simulink library "VRU_MC_Search"  (Simulink 8.1)
settings: Solver=ode1  StartTime=0.0  StopTime=Inf  FixedStep=0.001  RelTol=1e-3
PostLoadFcn:
  | , if any(exist('dsrtsu_mdlpostloadfcn', 'file') == [2, 3, 6]), try dsrtsu_mdlpostloadfcn('Execute', bdroot); catch fprintf('Error in PostLoadFcn (dsrtsu_mdlpostloadfcn) for model "%s":\n %s\n', bdroot, lasterr); end, end,
undefined symbols (not defined in the file or in its folder): KIFO_VRUExistProbLimit_num, ZERO_INT
settings Model: DSRTSU_INTERNAL_RTI_VER=450  DSRTSU_INTERNAL_RTI_TYPE=rti1401  RTICANMMDATA=struct('GeneralSetupData',struct('modelroot','D:\PROJECTS\HAITEC\TAIWAN_HAITEC_SVN\trunk\AdasDragon\software\sw_development\arch\app\ifo','generalsettings',struct('filesettings',struct('destfolder',struct('Name','RTICANMM_FILES','Check',1),'buildfolder',struct('Name','.','Check',1),'AbsDestfolder',struct('Name','D:\PROJECTS\HAITEC\TAIWAN_HAITEC_SVN\trunk\AdasDragon\software\sw_development\arch\app\ifo\RTICANMM_FILES'),'AbsBuildfolder',struct('Name','D:\PROJECTS\HAITEC\TAIWAN_HAITEC_SVN\trunk\AdasDragon\software\sw_development\arch\app\ifo'))),'options',struct('addpaths',1,'rmpaths',1,'addtrcexclusion',logical(1),'cannavigator',struct('checkmonitoring',0),'show_usrtrc',0,'use_usrtrc',0),'advanced',struct('options',[1 1 1 1 1 1 1 1 1 1 1 1 1 1 1 1 1 1 1 1 1 1 1 1 1 1 1 1 1 1 1 1 1 1 1 1 1 1 1 1 1 1 1 1 1 1 1 1 1 1 1 1 1 1 1 1 1 1 1 1 1 1 1 1 1 1 1 1 1 1 1 1 1 1 1 1 1 1 1 1 1 1 1 1 1 1 1 1 1 1 1 1 1 1 1 1 1 1 1 1]),'MPSetup',{{}},'modelname','VRU_MC_Search','block','VRU_MC_Search'))  DSRTSU_INTERNAL_RTIFPGA=40  Creator=tescamilla  LastModifiedBy=tescamilla

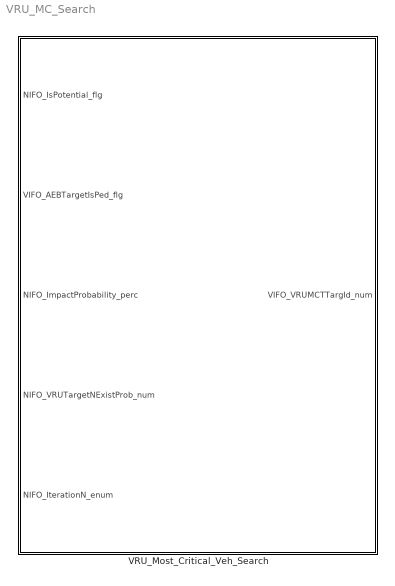
== system VRU_MC_Search ==
  VRU_Most_Critical_Veh_Search : Subsystem

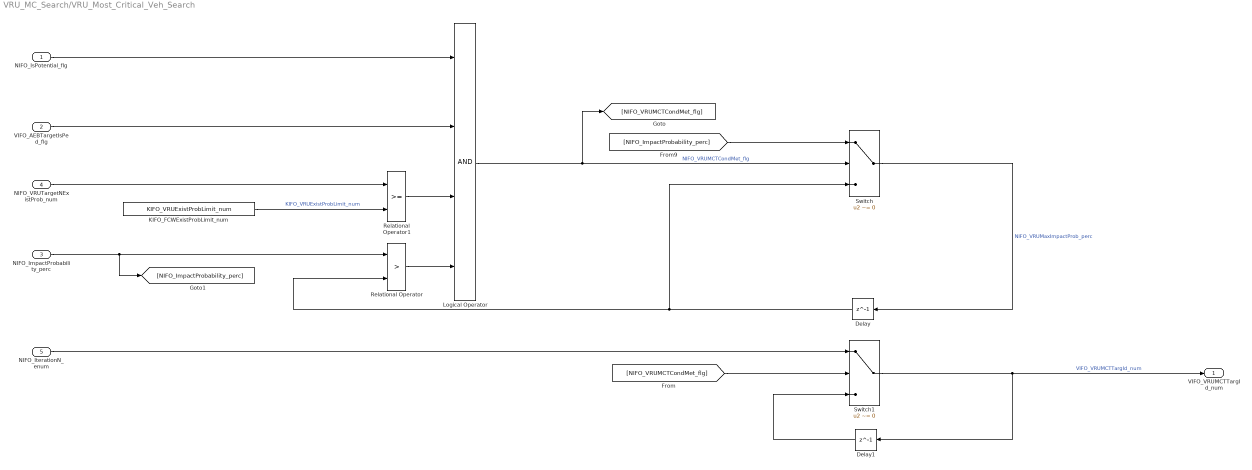
== system VRU_MC_Search/VRU_Most_Critical_Veh_Search ==
  NIFO_IsPotential_flg : Inport
  VIFO_AEBTargetIsPed_flg : Inport  Port=2
  NIFO_ImpactProbability_perc : Inport  Port=3
  NIFO_VRUTargetNExistProb_num : Inport  Port=4
  NIFO_IterationN_enum : Inport  Port=5
  Delay : Delay  DelayLength=1  InitialCondition=0
  Delay1 : Delay  DelayLength=1  InitialCondition=ZERO_INT
  KIFO_FCWExistProbLimit_num : Constant  Value=KIFO_VRUExistProbLimit_num
  Logical Operator : Logic  Inputs=4  AllPortsSameDT=off  OutDataTypeStr=boolean
  Relational Operator : RelationalOperator  Operator=>  OutDataTypeStr=boolean
  Relational Operator1 : RelationalOperator  OutDataTypeStr=boolean
  Switch : Switch  Criteria=u2 ~= 0
  Switch1 : Switch  Criteria=u2 ~= 0
  VIFO_VRUMCTTargId_num : Outport
  wires:
  NIFO_ImpactProbability_perc/1 -> [NIFO_ImpactProbability_perc], Relational Operator/1
  VIFO_AEBTargetIsPed_flg/1 -> Logical Operator/2
  NIFO_IsPotential_flg/1 -> Logical Operator/1
  Relational Operator/1 -> Logical Operator/4
  Delay/1 -> Relational Operator/2, Switch/3
  Delay1/1 -> Switch1/3
  Logical Operator/1 -> [NIFO_VRUMCTCondMet_flg], Switch/2  "NIFO_VRUMCTCondMet_flg"
  [NIFO_ImpactProbability_perc] -> Switch/1
  Switch1/1 -> VIFO_VRUMCTTargId_num/1, Delay1/1  "VIFO_VRUMCTTargId_num"
  Switch/1 -> Delay/1  "NIFO_VRUMaxImpactProb_perc"
  [NIFO_VRUMCTCondMet_flg] -> Switch1/2
  NIFO_IterationN_enum/1 -> Switch1/1
  NIFO_VRUTargetNExistProb_num/1 -> Relational Operator1/1
  KIFO_FCWExistProbLimit_num/1 -> Relational Operator1/2  "KIFO_VRUExistProbLimit_num"
  Relational Operator1/1 -> Logical Operator/3
